simulink model "LeadLag"  (R2021a)
settings: Solver=VariableStepAuto  StartTime=0.0  StopTime=50  RelTol=1e-3
libraries: simulink x1
settings Model: Creator=thibaut  LastModifiedBy=thibaut

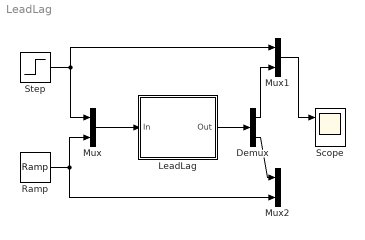
== system LeadLag ==
  Demux : Demux  Outputs=2
  LeadLag : Subsystem  mask{Ts=0.05, K_P=1, T_lag=3, T_lead=-1}
      mask prompts: Ts "Sampling period Ts [s]"; K_P "Process gain Kp"; T_lag "Lag time constant Tlag"; T_lead "Lead time constant Tlead"
  Mux : Mux  Inputs=2
  Mux1 : Mux  Inputs=2
  Mux2 : Mux  Inputs=2
  Ramp : simulink/Sources/Ramp  slope=1  start=0  InitialOutput=0
  Scope : Scope  NumInputPorts=2
  Step : Step  SampleTime=0.05
  wires:
  Step/1 -> Mux1/1, Mux/1
  Ramp/1 -> Mux2/2, Mux/2
  Mux/1 -> LeadLag/1(In)
  LeadLag/1(Out) -> Demux/1
  Demux/1 -> Mux1/2
  Demux/2 -> Mux2/1
  Mux1/1 -> Scope/1

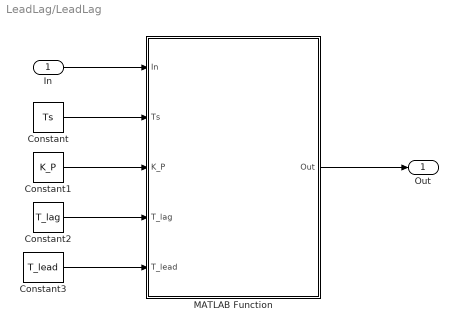
== system LeadLag/LeadLag ==
  In : Inport
  Constant : Constant  Value=Ts
  Constant1 : Constant  Value=K_P
  Constant2 : Constant  Value=T_lag
  Constant3 : Constant  Value=T_lead
  MATLAB Function : MATLAB Function  TreatAsAtomicUnit=on  SystemSampleTime=Ts
  Out : Outport
  wires:
  Constant3/1 -> MATLAB Function/5(T_lead)
  Constant1/1 -> MATLAB Function/3(K_P)
  MATLAB Function/1(Out) -> Out/1
  Constant2/1 -> MATLAB Function/4(T_lag)
  In/1 -> MATLAB Function/1(In)
  Constant/1 -> MATLAB Function/2(Ts)

== matlab function LeadLag/MATLAB Function ==
  data: In input; Out output; Ts input; K_P input; T_lag input; T_lead input
function Out = LeadLag(In,Ts,K_P,T_lag,T_lead)

persistent Out_p
persistent In_p

if isempty(Out_p)
    Out_p = K_P*In;
end

if isempty(In_p)
    In_p = 0*In;
end

% Euler backward
K = Ts/T_lag;
Out = (1/(1+K))*Out_p + ((K_P*K)/(1+K))*(((1+(T_lead/Ts))*In)-((T_lead/Ts)*In_p));
Out_p = Out;
In_p = In;
